simulink model "b_c"  (R2018a)
settings: Solver=FixedStepDiscrete  StartTime=0.0  StopTime=10  FixedStep=Ts  RelTol=1e-3
values from neighbouring files (symbols this model uses):
  Ts = 0.1    [Cal_input.m]
undefined symbols (not defined in the file or in its folder): tf_dlte2dtheta_d, tf_dlte2dtheta_full_d, tf_dlte2dtheta_half_d
settings Model: Creator=80741  LastModifiedBy=80741
settings DataIOCC: LimitDataPoints=on  SaveFormat=Array  SignalLoggingSaveFormat=ModelDataLogs
settings OptimizationCC: InitFltsAndDblsToZero=on  LifeSpan=inf
settings DebuggingCC: SaveWithParameterizedLinksMsg=none  UnderspecifiedInitializationDetection=Classic  MergeDetectMultiDrivingBlocksExec=none  SignalResolutionControl=TryResolveAllWithWarning  SolverPrmCheckMsg=warning  MultiTaskDSMMsg=warning  MultiTaskCondExecSysMsg=none  FcnCallInpInsideContextMsg=warning  SFUnexpectedBacktrackingDiag=warning  SFNoUnconditionalDefaultTransitionDiag=warning  SFExecutionAtInitializationDiag=none
settings HardwareCC: ProdBitPerPointer=32  ProdBitPerSizeT=32  ProdBitPerPtrDiffT=32  ProdLargestAtomicFloat=None  ProdIntDivRoundTo=Undefined  ProdEndianess=Unspecified  ProdWordSize=32  ProdHWDeviceType=32-bit Generic
settings ModelReferenceCC: PropagateSignalLabelsOutOfModel=off
settings CodeAppCC: StateflowObjectComments=on
settings GRTTargetCC: TargetFcnLib=ansi_tfl_tmw.mat  TargetLangStandard=C89/C90 (ANSI)  CombineOutputUpdateFcns=off  GRTInterface=on
settings ConfigComp: CovMetricSettings=dw  CovHtmlReporting=on  CovSaveCumulativeToWorkspaceVar=on  CovSaveSingleToWorkspaceVar=on  CovExternalEMLEnable=off

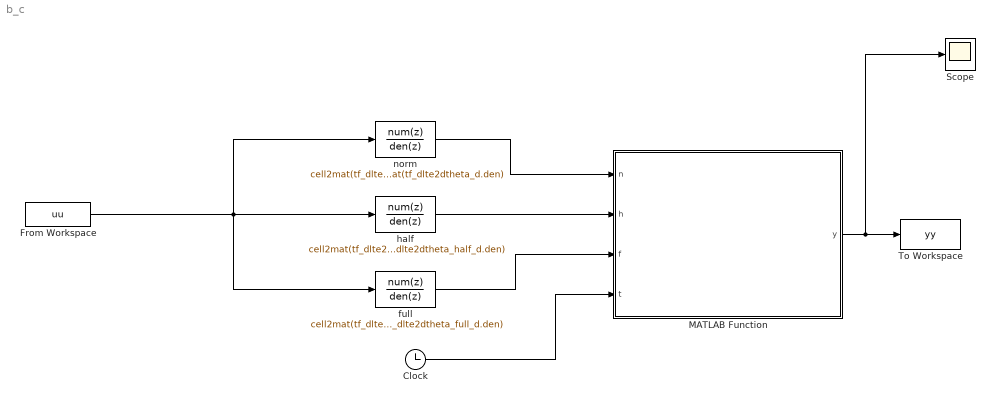
== system b_c ==
  Clock : Clock
  From Workspace : FromWorkspace  VariableName=uu  SampleTime=Ts
  MATLAB Function : MATLAB Function  TreatAsAtomicUnit=on
  Scope : Scope
  To Workspace : ToWorkspace  VariableName=yy  SaveFormat=Timeseries  SampleTime=-1
  full : DiscreteTransferFcn  Numerator=cell2mat(tf_dlte2dtheta_full_d.num)  Denominator=cell2mat(tf_dlte2dtheta_full_d.den)
  half : DiscreteTransferFcn  Numerator=cell2mat(tf_dlte2dtheta_half_d.num)  Denominator=cell2mat(tf_dlte2dtheta_half_d.den)
  norm : DiscreteTransferFcn  Numerator=cell2mat(tf_dlte2dtheta_d.num)  Denominator=cell2mat(tf_dlte2dtheta_d.den)
  wires:
  From Workspace/1 -> full/1, half/1, norm/1
  norm/1 -> MATLAB Function/1(n)
  half/1 -> MATLAB Function/2(h)
  full/1 -> MATLAB Function/3(f)
  Clock/1 -> MATLAB Function/4(t)
  MATLAB Function/1(y) -> Scope/1, To Workspace/1

== matlab function b_c/MATLAB Function ==
  data: n input; y output; h input; f input; t input
function y = fcn(n,h,f,t)
if(t>5)
    y=f;
elseif(t>2)
    y=h;
else
    y=n;
end
end
